simulink model "RealHardwareIoNull"  (R2015a)
settings: configuration reference "SIMULATION_CONFIGURATION" (kept outside this file)
settings Model: Creator=moritz  LastModifiedBy=moritz
settings ConfigSetRef: SourceLocation=Base Workspace

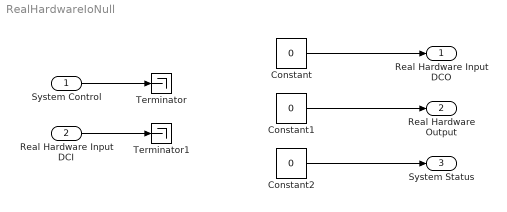
== system RealHardwareIoNull ==
  System Control : Inport  OutDataTypeStr=Bus: SYSTEM_CONTROL_BUS  BusOutputAsStruct=on
  Real Hardware Input DCI : Inport  Port=2  OutDataTypeStr=Bus: HARDWARE_IO_INPUT_BUS  BusOutputAsStruct=on
  Constant : Constant  Value=0  OutDataTypeStr=Bus: HARDWARE_IO_INPUT_BUS
  Constant1 : Constant  Value=0  OutDataTypeStr=Bus: HARDWARE_IO_OUTPUT_BUS
  Constant2 : Constant  Value=0  OutDataTypeStr=Bus: SYSTEM_STATUS_BUS
  Terminator : Terminator
  Terminator1 : Terminator
  Real Hardware Input DCO : Outport  OutDataTypeStr=Bus: HARDWARE_IO_INPUT_BUS  BusOutputAsStruct=on
  Real Hardware Output : Outport  Port=2  OutDataTypeStr=Bus: HARDWARE_IO_OUTPUT_BUS  BusOutputAsStruct=on
  System Status : Outport  Port=3  OutDataTypeStr=Bus: SYSTEM_STATUS_BUS  BusOutputAsStruct=on
  wires:
  Constant2/1 -> System Status/1
  Constant1/1 -> Real Hardware Output/1
  Constant/1 -> Real Hardware Input DCO/1
  Real Hardware Input DCI/1 -> Terminator1/1
  System Control/1 -> Terminator/1
